simulink model "PID_Model"  (R2022a)
settings: Solver=VariableStepAuto  StartTime=0.0  StopTime=10.0  RelTol=1e-3
values from neighbouring files (symbols this model uses):
  K = jacobian(eta, theta)    [stewart_jacobian_forward.m]
undefined symbols (not defined in the file or in its folder): La, Ra
settings Model: Creator=seungml  LastModifiedBy=seungml

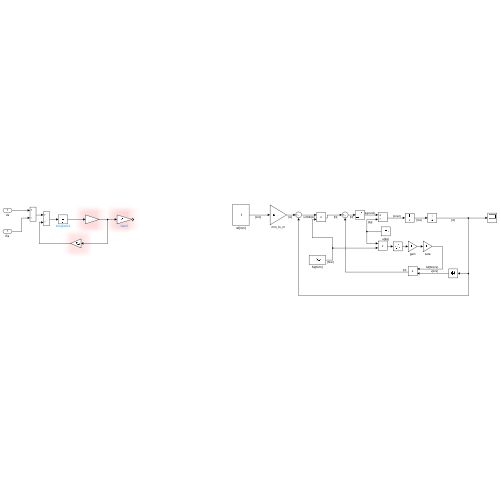
[thumbnail: Simulink's stored preview of the top-level diagram]
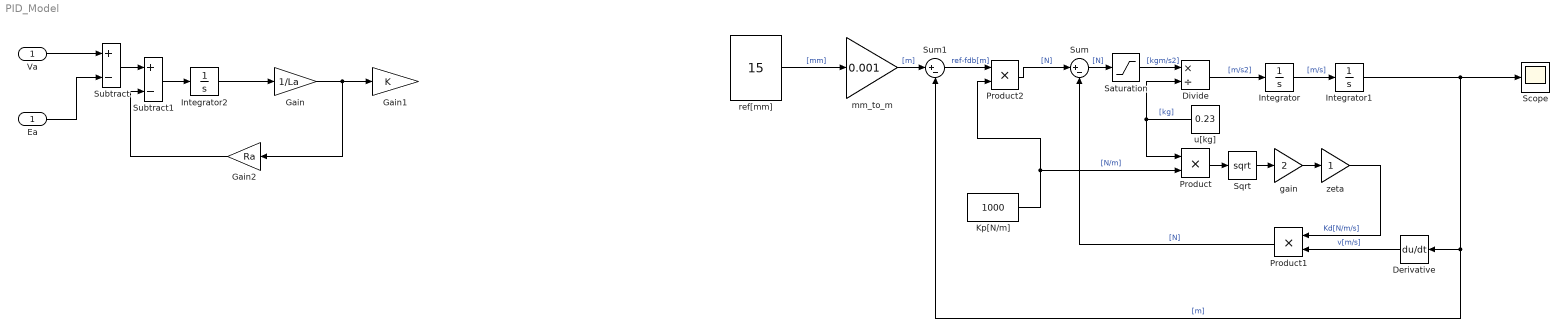
== system PID_Model ==
  Va : Inport
  Derivative : Derivative
  Divide : Product  Inputs=*/
  Ea : InportShadow
  Gain : Gain  Gain=1/La
  Gain1 : Gain  Gain=K
  Gain2 : Gain  Gain=Ra
  Integrator : Integrator
  Integrator1 : Integrator
  Integrator2 : Integrator
  Kp[N/m] : Constant  Value=1000
  Product : Product
  Product1 : Product
  Product2 : Product
  Saturation : Saturate  UpperLimit=22.3  LowerLimit=-22.3
  Scope : Scope
  Sqrt : Sqrt
  Subtract : Sum  Inputs=+-
  Subtract1 : Sum  Inputs=+-
  Sum : Sum  Inputs=|+-
  Sum1 : Sum  Inputs=|+-
  gain : Gain  Gain=2
  mm_to_m : Gain  Gain=0.001
  ref[mm] : Constant  Value=15
  u[kg] : Constant  Value=0.23
  zeta : Gain
  wires:
  Product2/1 -> Sum/1  "[N]"
  ref[mm]/1 -> mm_to_m/1  "[mm]"
  mm_to_m/1 -> Sum1/1  "[m]"
  Sum/1 -> Saturation/1  "[N]"
  Divide/1 -> Integrator/1  "[m/s2]"
  Integrator/1 -> Integrator1/1  "[m/s]"
  Integrator1/1 -> Scope/1, Derivative/1, Sum1/2  "[m]"
  Derivative/1 -> Product1/2  "v[m/s]"
  u[kg]/1 -> Product/1, Divide/2  "[kg]"
  Product/1 -> Sqrt/1
  Sqrt/1 -> gain/1
  gain/1 -> zeta/1
  zeta/1 -> Product1/1  "Kd[N/m/s]"
  Product1/1 -> Sum/2  "[N]"
  Sum1/1 -> Product2/1  "ref-fdb[m]"
  Kp[N/m]/1 -> Product/2, Product2/2  "[N/m]"
  Saturation/1 -> Divide/1  "[kgm/s2]"
  Va/1 -> Subtract/1
  Ea/1 -> Subtract/2
  Subtract/1 -> Subtract1/1
  Integrator2/1 -> Gain/1
  Gain/1 -> Gain1/1, Gain2/1
  Subtract1/1 -> Integrator2/1
  Gain2/1 -> Subtract1/2
